simulink model "s0906_3"  (Simulink 6.0)
settings: Solver=ode3  SolverMode=SingleTasking  StartTime=0.0  StopTime=900  FixedStep=1  MaxStep=1  RelTol=1e-3  AbsTol=1e-6
values from neighbouring files (symbols this model uses):
  T = 1    [m0304.m]
undefined symbols (not defined in the file or in its folder): rnend, rzaed, snend, szaed, wdachrad
settings Model: LastModifiedBy=Froriep
settings DataIOCC: LimitDataPoints=off  SaveOutput=off  TimeSaveName=t
settings OptimizationCC: BooleanDataType=off
settings DebuggingCC: SolverPrmCheckMsg=none
settings HardwareCC: TargetUnknown=on
settings STFCustomTargetCC: TargetFcnLib=ansi_tfl_tmw.mat  GenFloatMathFcnCalls=ANSI_C  ModelReferenceCompliant=off  SystemTargetFile=grt.tlc

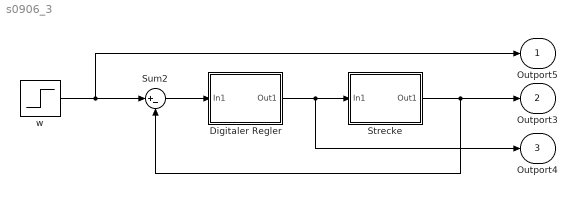
== system s0906_3 ==
  Digitaler Regler : Subsystem
      mask Display: disp('Gr(z)')
  Strecke : Subsystem
      mask Display: disp('Gs(z)')
  Sum2 : Sum  Inputs=|+-  SaturateOnIntegerOverflow=on  InputSameDT=on
  w : Step  Time=0  After=wdachrad  SampleTime=T
  Outport5 : Outport
  Outport3 : Outport  Port=2
  Outport4 : Outport  Port=3
  wires:
  w/1 -> Outport5/1, Sum2/1
  Digitaler Regler/1(Out1) -> Outport4/1, Strecke/1(In1)
  Strecke/1(Out1) -> Outport3/1, Sum2/2
  Sum2/1 -> Digitaler Regler/1(In1)

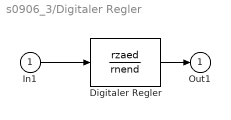
== system s0906_3/Digitaler Regler ==
  In1 : Inport  Port=1  LatchInput=off
  Digitaler Regler : DiscreteTransferFcn  Numerator=rzaed  Denominator=rnend  SampleTime=T
  Out1 : Outport
  wires:
  In1/1 -> Digitaler Regler/1
  Digitaler Regler/1 -> Out1/1

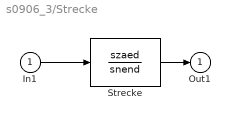
== system s0906_3/Strecke ==
  In1 : Inport  Port=1  LatchInput=off
  Strecke : DiscreteTransferFcn  Numerator=szaed  Denominator=snend  SampleTime=T
  Out1 : Outport
  wires:
  In1/1 -> Strecke/1
  Strecke/1 -> Out1/1
